simulink model "Optimal"  (R2016b)
settings: Solver=FixedStepAuto  StartTime=0.0  StopTime=tF  FixedStep=Ts  RelTol=1e-3
values from neighbouring files (symbols this model uses):
  k = 0.0001    [Proj_7.m]
  K_d = 0.2*sgn    [parameters.m]
  K_dth = 0.05    [Proj_1b.m]    (also in Proj_5.m = -0.04; parameters.m = 0.05*sgn)
  M_d = M_d_r(i)    [Proj_7.m]    (also in parameters.m = 200*sgn)
  T_m = 120    [parameters.m]
  tau = tau_i(i)    [Proj_4.m]    (also in parameters.m = 0.05)
settings Model: Creator=Daniel  LastModifiedBy=Daniel

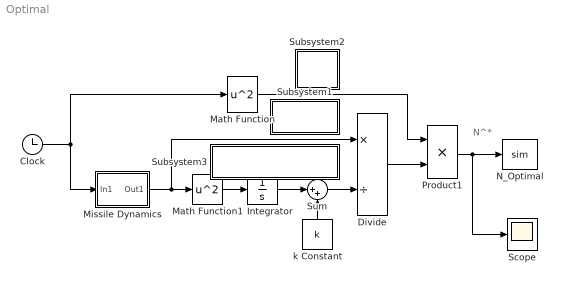
== system Optimal ==
  note: N^*
  Clock : Clock
  Divide : Product  Inputs=*/
  Integrator : Integrator
  Math Function : Math  Operator=square  SaturateOnIntegerOverflow=on
  Math Function1 : Math  Operator=square  SaturateOnIntegerOverflow=on
  Missile Dynamics : Subsystem
      mask Display: image('Gm_s.PNG');
  N_Optimal : ToWorkspace  VariableName=sim  SaveFormat=Timeseries  SampleTime=-1
  Product1 : Product
  Scope : Scope
  Subsystem1 : Subsystem
      mask Display: image('7_a.PNG');
  Subsystem2 : Subsystem
      mask Display: image('7_b.PNG');
  Subsystem3 : Subsystem
      mask Display: image('7_c.PNG');
  Sum : Sum  Inputs=|++
  k Constant : Constant  Value=k
  wires:
  Divide/1 -> Product1/2
  Sum/1 -> Divide/2
  k Constant/1 -> Sum/2
  Math Function/1 -> Product1/1
  Missile Dynamics/1(Out1) -> Math Function1/1, Divide/1
  Integrator/1 -> Sum/1
  Clock/1 -> Missile Dynamics/1(In1), Math Function/1
  Math Function1/1 -> Integrator/1
  Product1/1 -> Scope/1, N_Optimal/1

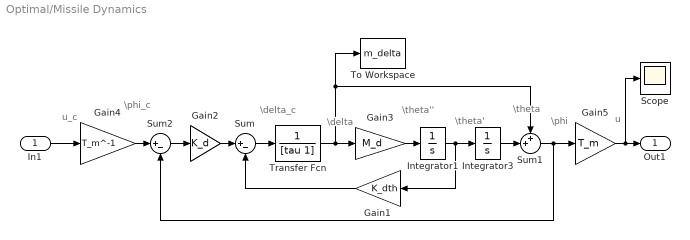
== system Optimal/Missile Dynamics ==
  note: \theta'
  note: \theta''
  note: \theta
  note: \delta
  note: \delta_c
  note: \phi_c
  note: \phi
  note: u
  note: u_c
  In1 : Inport
  Gain1 : Gain  Gain=K_dth
  Gain2 : Gain  Gain=K_d
  Gain3 : Gain  Gain=M_d
  Gain4 : Gain  Gain=T_m^-1
  Gain5 : Gain  Gain=T_m
  Integrator1 : Integrator
  Integrator3 : Integrator
  Scope : Scope
  Sum : Sum  Inputs=|+-
  Sum1 : Sum  Inputs=++|
  Sum2 : Sum  Inputs=|+-
  To Workspace : ToWorkspace  VariableName=m_delta  SaveFormat=Timeseries  SampleTime=-1
  Transfer Fcn : TransferFcn  Denominator=[tau 1]
  Out1 : Outport
  wires:
  Gain1/1 -> Sum/2
  Sum/1 -> Transfer Fcn/1
  Gain2/1 -> Sum/1
  Transfer Fcn/1 -> Sum1/1, To Workspace/1, Gain3/1
  Sum1/1 -> Sum2/2, Gain5/1
  Gain3/1 -> Integrator1/1
  Integrator1/1 -> Integrator3/1, Gain1/1
  Integrator3/1 -> Sum1/2
  Sum2/1 -> Gain2/1
  Gain5/1 -> Scope/1, Out1/1
  In1/1 -> Gain4/1
  Gain4/1 -> Sum2/1

== system Optimal/Subsystem1 ==

== system Optimal/Subsystem2 ==

== system Optimal/Subsystem3 ==
